simulink model "Clutchless_P2_Parallel"  (R2017b)
settings: Solver=FixedStepAuto  StartTime=0.0  StopTime=length(Speed)  FixedStep=0.01  MaxStep=0.01  RelTol=1e-3  EnableMultiTasking=on
PostLoadFcn:
  | , if any(exist('dsrtsu_mdlpostloadfcn', 'file') == [2, 3, 6]), try dsrtsu_mdlpostloadfcn('Execute', bdroot); catch fprintf('Error in PostLoadFcn (dsrtsu_mdlpostloadfcn) for model "%s":\n %s\n', bdroot, lasterr); end, end,
undefined symbols (not defined in the file): Actuators, APP1_OOR, APP2_OOR, APP_Mismatch, Brk_Flt, cal, Chassis, ClutchEngag, Clutchless_HSC, eng, Engine, EngineTorqueReal, EngOverTemp, ENGTRQ_MSMCH_Degraded_CP, ENGTRQ_MSMCH_ErrCritical_CP, ENGTRQ_MSMCH_LimpHome_CP, EngTrqMismatch, ess, ESSOverTemp, g, gb, Grade, KeyPos_Flt, lib_Actuators, lib_Chassis, lib_Clutchless_HSC, lib_EMachine_2017a, lib_Sensors_2017a, LossCAN, Machine, MCUOverTemp, mot, MotDirMismatch, motor_Trq, MotOverTemp, MotTrqMismatch, mph2ms, PRNDL_Flt, RegenFault, rho, Sensors, t_amb, time, tloop, veh, Vehicle
libraries: simulink x96, EC2_libraries x6, autolibmappedmotor x3, powerlib_meascontrol x2, CalculationGallon x1, lib_DCDC x1, lib_Differential x1, lib_HVESS x1, lib_Engine x1, lib_OBC x1, Scope_new x1, lib_Transmission x1
(part 3 of 10)

== system Clutchless_P2_Parallel/Camaro Plant Model/E-Machine/Soft MCU/Torque Calculation3 ==
  MotTrqReq : Inport
  MotSpd : Inport  Port=2
  MotTrqFdbck : Inport  Port=3
  Voltage : Inport  Port=4
  Abs : Abs  Commented=on  ZeroCross=off
  Abs1 : Abs  Commented=on  ZeroCross=off
  Mapped Generator : autolibmappedmotor/Mapped Motor  port_config=Speed  param_by=Maximum torque and power  w_t=[ 0 375 750 800 ]  T_t=[0.09 0.08 0.07 0]  torque_max=300  power_max=70000  Tc=0.02  param_loss=Tabulated efficiency data  eff=100  w_eff=375  T_eff=0.08  Piron=0  Pbase=0  w_eff_bp=[0 500 1000 1500 2000 2500 3000 3500 4000 4500 5000 5500 6000 6500 7000]  T_eff_bp=[25 50 75 100 112 125 150 165 175 200 225 250 262 275 300]  losses_table=[1.49 1.67 2.21 3.10; 0.42 0.69 1.14 2.03; 0.06 0.24 0.78 1.68; 0.42 0.69 1.14 2.03; 1.49 1.67 2.21 3.10]  efficiency_table=mot.plant.init.geneff_trq.map  J=5e-6  b=1e-5  omega_o=0  T_t_extended=[0 0.07 0.08 0.09 0.08 0.07 0]  w_t_extended=[-800 -750 -375 0 375 750 800]  KLossIron=0  KLossCopper=0  x_w_eff_vec=[-7000 -6500 -6000 -5500 -5000 -4500 -4000 -3500 -3000 -2500 -2000 -1500 -1000 -500 0 500 1000 1500 2000 2500 3000 3500 4000 4500 5000 5500 6000 6500 7000]  x_T_eff_vec=[-300 -275 -262 -250 -225 -200 -175 -165 -150 -125 -112 -100 -75 -50 -25 25 50 75 100 112 125 150 165 175 200 225 250 262 275 300]  x_losses_mat=[2566666.66666667 607894.736842105 517282.051282051 493589.743589743 393750 307317.073170732 233333.333333333 220000 200000 119318.181818182 106909.090909091 95454.5454545455 58333.3333333334 30434.7826086956 213888.888888889 96250 28000 52500 84000 94080 105000 168000 184800 196000 252000 315000 385000 403480 462000 1155000;2383333.33333333 290988.372093023 277232.558139535 221590.909090909 199431.818181818 144444.444444445 98913.0434782608 93260.8695652173 84782.6086956521 70652.1739130434 46468.085106383 41489.3617021276 42391.3043478261 28260.8695652174 198611.111111111 89375 26000 39000 39000 43680 65000 78000 85800 91000 130000 175500 195000 238420 250250 1072500;2200000 183333.333333333 174666.666666667 166666.666666667 150000 76595.744680851 67021.2765957447 63191.4893617021 57446.8085106383 47872.3404255319 42893.6170212766 38297.8723404255 50000 40909.0909090909 183333.333333333 82500 36000 45000 36000 40320 45000 53999.9999999999 59399.9999999999 62999.9999999999 71999.9999999999 135000 150000 157200 165000 990000;2016666.66666667 96542.5531914893 91978.7234042553 87765.9574468085 78989.3617021276 70212.7659574468 61436.1702127659 57925.5319148936 52659.5744680851 43882.9787234042 39319.1489361702 35106.3829787234 45833.3333333334 37500 168055.555555556 75625 33000 41250 33000 36960 41250 49499.9999999999 54449.9999999999 57749.9999999999 65999.9999999999 74249.9999999999 82499.9999999999 86459.9999999999 90749.9999999999 907500;1833333.33333333 87765.9574468085 83617.0212765957 79787.2340425532 71808.5106382979 63829.7872340425 55851.0638297872 52659.5744680851 47872.3404255319 39893.6170212766 35744.6808510638 109756.097560976 41666.6666666667 34090.9090909091 152777.777777778 68750 30000 37500 90000 33600 37500 45000 49499.9999999999 52499.9999999999 59999.9999999999 67499.9999999999 74999.9999999999 78599.9999999999 82499.9999999999 825000;1650000 78989.3617021276 75255.3191489361 71808.5106382979 64627.6595744681 57446.8085106383 50265.9574468085 47393.6170212766 43085.1063829787 35904.2553191489 43826.0869565217 50000 46022.7272727273 36627.9069767442 137500 61875 31500 40500 45000 40320 33750 40500 44550 47250 53999.9999999999 60749.9999999999 67499.9999999999 70739.9999999999 74249.9999999999 742500;1466666.66666667 733333.333333333 698666.666666667 86956.5217391304 57446.8085106383 51063.829787234 44680.8510638298 42127.6595744681 52173.9130434782 43478.2608695652 49777.7777777778 44444.4444444445 48837.2093023256 50000 122222.222222222 55000 40000 42000 40000 44800 40000 48000 39600 42000 48000 53999.9999999999 80000 419200 440000 660000;1283333.33333333 641666.666666667 611333.333333333 97222.2222222223 50265.9574468085 44680.8510638298 53260.8695652174 50217.3913043478 45652.1739130435 48611.1111111111 43555.5555555556 47727.2727272728 57621.9512195122 49358.9743589743 106944.444444444 48125 38500 47250 42000 39200 43750 42000 46200 49000 42000 47250 87500 366800 385000 577500;1100000 550000 524000 500000 75000 38297.8723404255 45652.1739130435 43043.4782608695 39130.4347826087 41666.6666666667 37333.3333333334 33333.3333333334 52777.7777777778 42307.6923076923 91666.6666666667 41250 33000 42750 30000 33600 37500 36000 39600 42000 36000 67500 300000 314400 330000 495000;916666.666666667 458333.333333333 436666.666666667 416666.666666667 375000 333333.333333333 27925.5319148936 35869.5652173913 32608.6956521739 34722.2222222222 31111.1111111111 40697.6744186047 43981.4814814815 39473.6842105263 76388.8888888889 34375 30000 35625 35000 28000 31250 30000 33000 26250 200000 225000 250000 262000 275000 412500;733333.333333333 366666.666666667 349333.333333333 333333.333333333 300000 266666.666666667 233333.333333333 45000 19148.9361702128 27777.7777777778 24888.8888888889 38095.2380952381 35185.1851851852 35135.1351351351 61111.1111111111 27500 26000 28500 32000 22400 25000 18000 39600 140000 160000 180000 200000 209600 220000 330000;550000 275000 262000 250000 225000 200000 175000 15797.8723404255 ...(+5787 chars)]
      settings: SourceProductName=Powertrain Blockset  SourceProductBaseCode=PW
  Mapped Motor : autolibmappedmotor/Mapped Motor  port_config=Speed  param_by=Maximum torque and power  w_t=[ 0 375 750 800 ]  T_t=[0.09 0.08 0.07 0]  torque_max=337  power_max=80000  Tc=0.02  param_loss=Tabulated efficiency data  eff=100  w_eff=375  T_eff=0.08  Piron=0  Pbase=0  w_eff_bp=[0 500 1000 1500 2000 2500 3000 3500 4000 4500 5000 5500 6000 6500 7000]  T_eff_bp="[88.2  98.7 106.4 119 132.2 155.6 175.6 208 243 295.3 328 329 333.5 334.5 335]"  losses_table=[1.49 1.67 2.21 3.10; 0.42 0.69 1.14 2.03; 0.06 0.24 0.78 1.68; 0.42 0.69 1.14 2.03; 1.49 1.67 2.21 3.10]  efficiency_table=mot.plant.init.moteff_trq.map  J=5e-6  b=1e-5  omega_o=0  T_t_extended=[0 0.07 0.08 0.09 0.08 0.07 0]  w_t_extended=[-800 -750 -375 0 375 750 800]  KLossIron=0  KLossCopper=0  x_w_eff_vec=[-7000 -6500 -6000 -5500 -5000 -4500 -4000 -3500 -3000 -2500 -2000 -1500 -1000 -500 0 500 1000 1500 2000 2500 3000 3500 4000 4500 5000 5500 6000 6500 7000]  x_T_eff_vec=[-335 -334.5 -333.5 -329 -328 -295.3 -243 -208 -175.6 -155.6 -132.2 -119 -106.4 -98.7 -88.2 88.2 98.7 106.4 119 132.2 155.6 175.6 208 243 295.3 328 329 333.5 334.5 335]  x_losses_mat=[1563333.33333333 381174.418604651 318340.909090909 314045.454545455 313090.909090909 281877.272727273 231954.545454546 161777.777777778 136577.777777778 94713.0434782608 80469.5652173912 72434.7826086956 31033.3333333334 60078.2608695652 411600 246960 55272 29792 66640 74032 87136 122920 145600 204120 248052 275520 276360 280140 327810 938000;1451666.66666667 296488.636363637 240861.111111111 185956.52173913 185391.304347826 166908.695652174 137347.826086956 117565.217391304 99252.1739130434 87947.8260869565 74721.7391304347 85944.4444444445 94309.090909091 104438.372093023 382200 229320 89817 82992 77350 68744 80912 91312 108160 126360 153556 170560 171080 216775 260910 871000;1340000 273681.818181818 222333.333333333 171652.173913043 171130.434782609 73825.0000000001 126782.608695652 108521.739130435 91617.3913043478 81182.6086956521 68973.9130434782 79333.3333333334 87054.5454545455 96404.6511627907 352800 211680 82908 76608 71400 63456 74688 84288 99840 116640 70872.0000000001 157440 157920 200100 240840 804000;1228333.33333333 1226500 203805.555555556 157347.826086956 115148.936170213 67672.9166666668 55687.5000000001 73021.2765957447 83982.6086956521 74417.3913043478 63226.0869565217 72722.2222222222 79800.0000000001 88370.9302325582 323400 194040 75999 70224 65450 58168 68464 77264 68639.9999999999 53460.0000000001 64966.0000000001 108240 144760 183425 735900 737000;1116666.66666667 1115000 1111666.66666667 182777.777777778 104680.85106383 61520.8333333334 50625.0000000001 66382.9787234042 56042.5531914893 67652.1739130434 57478.2608695652 66111.1111111111 72545.4545454546 80337.2093023256 294000 176400 69090 63840 59500 52880 62240 52679.9999999999 62399.9999999999 48600 59060.0000000001 98399.9999999999 164500 667000 669000 670000;1005000 1003500 1000500 987000 984000 115552.173913043 95086.9565217391 81391.304347826 68713.0434782608 60886.9565217391 66100 59500 65290.9090909091 97496.3414634146 264600 158760 79947 57456 53550 59490 56016 63216 74880 87480 106308 590400 592200 600300 602100 603000;893333.333333333 892000 889333.333333333 877333.333333333 145777.777777778 131244.444444445 84521.7391304347 72347.8260869565 61078.2608695652 54121.7391304347 58755.5555555556 58831.4606741573 69283.7209302326 98700 235200 141120 78960 59584 52360 52880 49792 56192 66560 77760 118120 131200 526400 533600 535200 536000;781666.666666667 780500 778166.666666667 767666.666666667 765333.333333333 689033.333333333 567000 485333.333333333 53443.4782608695 60511.1111111111 57187.6404494382 56795.4545454546 70933.3333333333 97434.6153846153 205800 123480 75999 59584 49980 50897 54460 49168 291200 340200 413420 459200 460600 466900 468300 469000;670000 669000 667000 658000 656000 590600 486000 416000 351200 51866.6666666667 49017.9775280899 58116.2790697675 65378.313253012 93505.2631578948 176400 105840 71064 54264 49980 43626 46680 210720 249600 291600 354360 393600 394800 400200 401400 402000;558333.333333333 557500 555833.333333333 548333.333333333 546666.666666667 492166.666666667 405000 346666.666666667 292666.666666667 259333.333333333 53802.3255813954 56666.6666666667 62395.061728395 110858.695652174 147000 88200 76492.5 50540 47600 46270 155600 175600 208000 243000 295300 328000 329000 333500 334500 335000;446666.666666667 446000 444666.666666667 438666.666666667 437333.333333333 393733.333333333 324000 277333.333333333 234133.333333333 207466.666666667 43041.8604651163 45333.3333333333 60020.5128205128 88686.9565217391 117600 70560 61194 46816 38080 37016 124480 140480 166400 194400 236240 262400 263200 266800 267600 268000;335000 334500 333500 329000 328000 295300 243000 208000 175600 155600 32281.3953488372 34000 50400 79719.2307692308 88200 52920 51817.5 38304 28560 27762 93360 105360 124800 145800 177180 196800 197400 200100 200700 201000;223333.333333333 223000 222333.333333333 219333.333333333 218666.666666667 196866.666666667 162000 138666.666666667 117066.666666667 103733.333333333 21520.9302325581 22666.6666666667 ...(+4913 chars)]
      settings: SourceProductName=Powertrain Blockset  SourceProductBaseCode=PW
  Mapped Motor1 : autolibmappedmotor/Mapped Motor  Commented=on  port_config=Torque  param_by=Maximum torque and power  w_t=[ 0 375 750 800 ]  T_t=[0.09 0.08 0.07 0]  torque_max=337  power_max=70000  Tc=0.02  param_loss=Tabulated efficiency data  eff=100  w_eff=375  T_eff=0.08  Piron=0  Pbase=0  w_eff_bp=[0 500 1000 1500 2000 2500 3000 3500 4000 4500 5000 5500 6000 6500 7000]  T_eff_bp="[88.2  98.7 106.4 119 132.2 155.6 175.6 208 243 295.3 328 329 333.5 334.5 335]"  losses_table=[1.49 1.67 2.21 3.10; 0.42 0.69 1.14 2.03; 0.06 0.24 0.78 1.68; 0.42 0.69 1.14 2.03; 1.49 1.67 2.21 3.10]  efficiency_table=mot.plant.init.moteff_trq.map  J=5e-6  b=1e-5  omega_o=0  T_t_extended=[0 0.07 0.08 0.09 0.08 0.07 0]  w_t_extended=[-800 -750 -375 0 375 750 800]  KLossIron=0  KLossCopper=0  x_w_eff_vec=[-7000 -6500 -6000 -5500 -5000 -4500 -4000 -3500 -3000 -2500 -2000 -1500 -1000 -500 0 500 1000 1500 2000 2500 3000 3500 4000 4500 5000 5500 6000 6500 7000]  x_T_eff_vec=[-335 -334.5 -333.5 -329 -328 -295.3 -243 -208 -175.6 -155.6 -132.2 -119 -106.4 -98.7 -88.2 88.2 98.7 106.4 119 132.2 155.6 175.6 208 243 295.3 328 329 333.5 334.5 335]  x_losses_mat=[1563333.33333333 381174.418604651 318340.909090909 314045.454545455 313090.909090909 281877.272727273 231954.545454546 161777.777777778 136577.777777778 94713.0434782608 80469.5652173912 72434.7826086956 31033.3333333334 60078.2608695652 411600 246960 55272 29792 66640 74032 87136 122920 145600 204120 248052 275520 276360 280140 327810 938000;1451666.66666667 296488.636363637 240861.111111111 185956.52173913 185391.304347826 166908.695652174 137347.826086956 117565.217391304 99252.1739130434 87947.8260869565 74721.7391304347 85944.4444444445 94309.090909091 104438.372093023 382200 229320 89817 82992 77350 68744 80912 91312 108160 126360 153556 170560 171080 216775 260910 871000;1340000 273681.818181818 222333.333333333 171652.173913043 171130.434782609 73825.0000000001 126782.608695652 108521.739130435 91617.3913043478 81182.6086956521 68973.9130434782 79333.3333333334 87054.5454545455 96404.6511627907 352800 211680 82908 76608 71400 63456 74688 84288 99840 116640 70872.0000000001 157440 157920 200100 240840 804000;1228333.33333333 1226500 203805.555555556 157347.826086956 115148.936170213 67672.9166666668 55687.5000000001 73021.2765957447 83982.6086956521 74417.3913043478 63226.0869565217 72722.2222222222 79800.0000000001 88370.9302325582 323400 194040 75999 70224 65450 58168 68464 77264 68639.9999999999 53460.0000000001 64966.0000000001 108240 144760 183425 735900 737000;1116666.66666667 1115000 1111666.66666667 182777.777777778 104680.85106383 61520.8333333334 50625.0000000001 66382.9787234042 56042.5531914893 67652.1739130434 57478.2608695652 66111.1111111111 72545.4545454546 80337.2093023256 294000 176400 69090 63840 59500 52880 62240 52679.9999999999 62399.9999999999 48600 59060.0000000001 98399.9999999999 164500 667000 669000 670000;1005000 1003500 1000500 987000 984000 115552.173913043 95086.9565217391 81391.304347826 68713.0434782608 60886.9565217391 66100 59500 65290.9090909091 97496.3414634146 264600 158760 79947 57456 53550 59490 56016 63216 74880 87480 106308 590400 592200 600300 602100 603000;893333.333333333 892000 889333.333333333 877333.333333333 145777.777777778 131244.444444444 84521.7391304347 72347.8260869565 61078.2608695652 54121.7391304347 58755.5555555556 58831.4606741573 69283.7209302326 98700 235200 141120 78960 59584 52360 52880 49792 56192 66560 77760 118120 131200 526400 533600 535200 536000;781666.666666667 780500 778166.666666667 767666.666666667 765333.333333333 689033.333333333 567000 485333.333333333 53443.4782608695 60511.1111111111 57187.6404494382 56795.4545454546 70933.3333333333 97434.6153846153 205800 123480 75999 59584 49980 50897 54460 49168 291200 340200 413420 459200 460600 466900 468300 469000;670000 669000 667000 658000 656000 590600 486000 416000 351200 51866.6666666667 49017.9775280899 58116.2790697675 65378.313253012 93505.2631578948 176400 105840 71064 54264 49980 43626 46680 210720 249600 291600 354360 393600 394800 400200 401400 402000;558333.333333333 557500 555833.333333333 548333.333333333 546666.666666667 492166.666666667 405000 346666.666666667 292666.666666667 259333.333333333 53802.3255813954 56666.6666666667 62395.061728395 110858.695652174 147000 88200 76492.5 50540 47600 46270 155600 175600 208000 243000 295300 328000 329000 333500 334500 335000;446666.666666667 446000 444666.666666667 438666.666666667 437333.333333333 393733.333333333 324000 277333.333333333 234133.333333333 207466.666666667 43041.8604651163 45333.3333333333 60020.5128205128 88686.9565217391 117600 70560 61194 46816 38080 37016 124480 140480 166400 194400 236240 262400 263200 266800 267600 268000;335000 334500 333500 329000 328000 295300 243000 208000 175600 155600 32281.3953488372 34000 50400 79719.2307692308 88200 52920 51817.5 38304 28560 27762 93360 105360 124800 145800 177180 196800 197400 200100 200700 201000;223333.333333333 223000 222333.333333333 219333.333333333 218666.666666667 196866.666666667 162000 138666.666666667 117066.666666667 103733.333333333 21520.9302325581 22666.6666666667 ...(+4913 chars)]
      settings: SourceProductName=Powertrain Blockset  SourceProductBaseCode=PW
  MinMax : MinMax  Commented=on  Inputs=2  ZeroCross=off
  MotSpd1 : InportShadow  Port=2
  MotTrqReq1 : InportShadow
  Product : Product  Commented=on
  Scope : Scope  Commented=on
  Scope1 : Scope  Commented=on
  Scope2 : Scope  Commented=on
  Sign : Signum  Commented=on  ZeroCross=off
  Subsystem : Subsystem
  Subsystem1 : Subsystem
  Terminator : Terminator
  Terminator1 : Terminator
  Terminator3 : Terminator
  "max torque " : Subsystem  Commented=on
  current : Outport
  mot_trq_out1 : Outport  Port=2
  wires:
  "max torque "/1(max torque) -> Abs1/1
  MotSpd/1 -> "max torque "/2(speed)
  MotTrqReq/1 -> Sign/1, Abs/1, "max torque "/1(Req)
  Sign/1 -> Product/1
  MinMax/1 -> Product/2
  Abs/1 -> MinMax/1
  Abs1/1 -> MinMax/2
  MotTrqFdbck/1 -> "max torque "/3(torque)
  MotTrqReq1/1 -> Mapped Generator/3, Subsystem1/2(In2), Subsystem/2(In2), Mapped Motor1/2, Mapped Motor/3
  MotSpd1/1 -> Mapped Generator/2, Mapped Motor/2
  Voltage/1 -> Mapped Motor1/1, Mapped Generator/1, Mapped Motor/1
  Mapped Motor/1 -> Terminator/1
  Mapped Generator/1 -> Terminator1/1
  Mapped Motor/3 -> Subsystem/1(In1)
  Mapped Generator/3 -> Subsystem/3(In3)
  Mapped Motor/2 -> Subsystem1/1(In1)
  Mapped Generator/2 -> Subsystem1/3(In3)
  Subsystem/1(Torq) -> mot_trq_out1/1
  Subsystem1/1(Current) -> current/1
  Mapped Motor1/3 -> Scope1/1
  Mapped Motor1/2 -> Scope2/1
  Mapped Motor1/1 -> Terminator3/1
  Mapped Motor1/4 -> Scope/1

== system Clutchless_P2_Parallel/Camaro Plant Model/Scopes/AxlTrq_to_EngTrq2/Ratio Filter ==
  Ratio : Inport
  Abs : Abs
  Compare To Zero : simulink/Logic and Bit Operations/Compare To Zero  relop===  OutDataTypeStr=boolean
  Constant : Constant  Value=cal.Time.TrnsOvrllEstTrqRatioSwitch
  Mature_Delay : EC2_libraries/Mature_Delay
      settings: SourceProductName=The database C:\Users\vrajm\AppData\Roaming\MathWorks\MATLAB\R2017b\slblocks_master.db is locked, or a table in the database is locked. (database is locked)
  Memory1 : Memory  InitialCondition=1
  Switch1 : Switch  Threshold=1
  Switch2 : Switch  Threshold=1
  Filtered_Ratio : Outport
  wires:
  Ratio/1 -> Compare To Zero/1, Abs/1
  Compare To Zero/1 -> Mature_Delay/1, Switch2/2
  Abs/1 -> Switch1/1, Switch2/3
  Switch1/1 -> Switch2/1
  Constant/1 -> Mature_Delay/2
  Mature_Delay/1 -> Switch1/2
  Memory1/1 -> Switch1/3
  Switch2/1 -> Filtered_Ratio/1, Memory1/1  "gear_ratio"

== system Clutchless_P2_Parallel/Camaro Plant Model/Scopes/AxlTrq_to_MtrTrq2/Ratio Filter ==
  Ratio : Inport
  Abs : Abs
  Compare To Zero : simulink/Logic and Bit Operations/Compare To Zero  relop===  OutDataTypeStr=boolean
  Constant : Constant  Value=cal.Time.TrnsOvrllEstTrqRatioSwitch
  Mature_Delay : EC2_libraries/Mature_Delay
      settings: SourceProductName=The database C:\Users\vrajm\AppData\Roaming\MathWorks\MATLAB\R2017b\slblocks_master.db is locked, or a table in the database is locked. (database is locked)
  Memory1 : Memory  InitialCondition=1
  Switch1 : Switch  Threshold=1
  Switch2 : Switch  Threshold=1
  Filtered_Ratio : Outport
  wires:
  Ratio/1 -> Compare To Zero/1, Abs/1
  Compare To Zero/1 -> Mature_Delay/1, Switch2/2
  Abs/1 -> Switch1/1, Switch2/3
  Switch1/1 -> Switch2/1
  Constant/1 -> Mature_Delay/2
  Mature_Delay/1 -> Switch1/2
  Memory1/1 -> Switch1/3
  Switch2/1 -> Filtered_Ratio/1, Memory1/1  "gear_ratio"

== system Clutchless_P2_Parallel/Clutchless_HSC/HSC/Camaro Fault Detection/Component Diagnostic ==
  note: Component Status Setting Rule
      | xxx_CompStatus could be 0, 1, 2 or 3
      | 0: component needs to be offline
      | 1: component needs torque plant to deliver creep torque
      | 2: component needs torque plant to limit maximum torque delivery
      | 3: component needs torque plant to operate normally
  note: Component Diagnostics
  SignalDiag : Inport
  Bus Creator : BusCreator  Inputs=6
  Driver Input Diagnostic : Subsystem
  ESS Component Diagnostic : Subsystem
  Engine Component Diagnostic : Subsystem
  Override Driver Status : Subsystem
  Override ESS Status : Subsystem
  Override Engine Status : Subsystem
  Override TCM Status : Subsystem
  Transmission Component Diagnostic : Subsystem
  CompDiag : Outport
  wires:
  SignalDiag/1 -> Engine Component Diagnostic/1(In1), Transmission Component Diagnostic/1(In1), Bus Creator/6, ESS Component Diagnostic/1(In1), Driver Input Diagnostic/1(In1)  "RawSig"
  Bus Creator/1 -> CompDiag/1
  Driver Input Diagnostic/1(Out1) -> Override Driver Status/1(In1)  "Diver_CompDiag"
  ESS Component Diagnostic/1(Out1) -> Override ESS Status/1(In1)  "ESS_CompDiag"
  Engine Component Diagnostic/1(Out1) -> Override Engine Status/1(In1)  "ECM_CompDiag"
  Transmission Component Diagnostic/1(Out1) -> Override TCM Status/1(In1)  "TCM_CompDiag"
  Override ESS Status/1(Out1) -> Bus Creator/2  "BMS_Status"
  Override Engine Status/1(Out1) -> Bus Creator/3  "ECM_Status"
  Override TCM Status/1(Out1) -> Bus Creator/5  "TCM_Status"
  Override Driver Status/1(Out1) -> Bus Creator/1  "Driver_Input_Status"
  Engine Component Diagnostic/2(Out2) -> Bus Creator/4  "EngTrqMismchType"

== system Clutchless_P2_Parallel/Clutchless_HSC/HSC/Camaro Fault Detection/Input Conversions ==
  note: Input Conversions and Override Switches
  note: These subsystems convert variable types to match those used in the
      | supervisor. In addition, override switches installed on each signal can
      | be used to manually override and signal for testing purposes
  RawSig : Inport
  BMS_Conversions : Subsystem
  Bus Creator : BusCreator  Inputs=5
  DriverInput_Conversions : Subsystem
  ECM_Conversions : Subsystem
  TCM_Conversions : Subsystem
  VehSig : Outport
  wires:
  DriverInput_Conversions/1(Out1) -> Bus Creator/1
  Bus Creator/1 -> VehSig/1  "InputConvAndOvrd"
  BMS_Conversions/1(Out1) -> Bus Creator/2
  RawSig/1 -> DriverInput_Conversions/1(In1), Bus Creator/5, TCM_Conversions/1(In1), ECM_Conversions/1(In1), BMS_Conversions/1(In1)  "RawSig"
  ECM_Conversions/1(Out1) -> Bus Creator/3
  TCM_Conversions/1(Out1) -> Bus Creator/4

== system Clutchless_P2_Parallel/Clutchless_HSC/HSC/Camaro Fault Detection/Signal Diagnostic ==
  note: These subsystems evaluate each signal for proper value range and other checks
  note: Signal Diagnostics
  VehSig : Inport
  Bus Creator : BusCreator  Inputs=5
  Driver Signal Diagnostic : Subsystem
  ESS Signal Diagnostic : Subsystem
  Engine Signal Diagnostic : Subsystem
  Subsystem1 : Subsystem
      mask Display: fprintf('Signal Naming Rule')
  Transmission Signal Diagnostic : Subsystem
  SignalDiag : Outport
  wires:
  VehSig/1 -> ESS Signal Diagnostic/1(Sensors1), Driver Signal Diagnostic/1(Sensors1), Engine Signal Diagnostic/1(Sensors1), Bus Creator/5, Transmission Signal Diagnostic/1(Sensors1)
  Driver Signal Diagnostic/1(Driver_SigDiag) -> Bus Creator/1  "Driver_SigDiag"
  ESS Signal Diagnostic/1(ESS_SigDiag) -> Bus Creator/2  "ESS_SigDiag"
  Engine Signal Diagnostic/1(Engine_SigDiag) -> Bus Creator/3  "Engine_SigDiag"
  Transmission Signal Diagnostic/1(Out2) -> Bus Creator/4  "Transmission_SigDiag"
  Bus Creator/1 -> SignalDiag/1  "SignalDiag"

== system Clutchless_P2_Parallel/Clutchless_HSC/HSC/Driver_Requests/APP_BPP to DrvIntndAxlTrq2 ==
  note: $Author: fy6949 $
      | $Rev: 577 $
      | $Date: 2017-1-19 08:53:15 -0500  $
  note: Note:Driver requested Axle Torque Calculation
  Sensors : Inport
  Diag : Inport  Port=2
  Controls : Inport  Port=3
  Bus Selector : BusSelector  OutputSignals=from_Analog.Driver_APP1,from_CAN.fromVEH_CAN.from_BCM.BrkPdlPos,from_CAN.fromEBCAN.from_ECM.VehSpdAvgDrvn,from_CAN.fromVEH_CAN.from_TCM.TrnGrRat,from_CAN.fromHV_CAN.from_MCU.INV_VCU_01.INV_Speed
  Bus Selector1 : BusSelector  OutputSignals=CompSig.RawSig.Driver_SigDiag.Drv_APP_Agree
  Bus Selector2 : BusSelector  OutputSignals=mode
  Post Driver Intnded Axle Torque : Subsystem
  Terminator : Terminator
  Terminator1 : Terminator
  IntndAxlTrq : Outport
  wires:
  Bus Selector2/1 -> Post Driver Intnded Axle Torque/5(Mode)  "<mode>"
  Bus Selector1/1 -> Terminator1/1  "<Drv_APP_Agree>"
  Diag/1 -> Bus Selector1/1
  Post Driver Intnded Axle Torque/2(BrkIntndAxlTrq) -> Terminator/1
  Bus Selector/1 -> Post Driver Intnded Axle Torque/1(APP)  "<Driver_APP1>"
  Bus Selector/4 -> Post Driver Intnded Axle Torque/4(TransGearRatio)  "<TrnGrRat>"
  Bus Selector/5 -> Post Driver Intnded Axle Torque/6(Motor_Speed)  "<INV_Speed>"
  Bus Selector/3 -> Post Driver Intnded Axle Torque/3(VehicleSpeed)  "<VehSpdAvgDrvn>"
  Bus Selector/2 -> Post Driver Intnded Axle Torque/2(BPP)  "<BrkPdlPos>"
  Post Driver Intnded Axle Torque/1(IntndAxlTrq) -> IntndAxlTrq/1
  Controls/1 -> Bus Selector2/1
  Sensors/1 -> Bus Selector/1

== system Clutchless_P2_Parallel/Clutchless_HSC/HSC/Powertrain Manager/HV Manager ==
  Sensors : Inport
  Controls : Inport  Port=2
  Axiomatic_Output_Manager : Subsystem
  BMS_Manager : Subsystem
  Bus Creator1 : BusCreator  Inputs=4
  DCDC Manager : Subsystem
  Inverter Manager : Subsystem
  OBC_Manager : Subsystem
  BMS_CAN : Outport
  HV_BUS_Status : Outport  Port=2
  OBC_CAN : Outport  Port=3
  OBC_Digital : Outport  Port=4
  BMS_Digital : Outport  Port=5
  Axiomatic_CAN : Outport  Port=6
  tag scope: MCU_CAN=global
  wires:
  [MCU_Status] -> BMS_Manager/3(In1)
  DCDC Manager/1(Out1) -> Bus Creator1/4
  Inverter Manager/3(MCU_Relay) -> Bus Creator1/3  "MCU_Relay"
  Axiomatic_Output_Manager/1(Axiomatic_CAN) -> Axiomatic_CAN/1
  BMS_Manager/3(BMS Digital) -> BMS_Digital/1
  BMS_Manager/1(BMS CAN) -> BMS_CAN/1
  Controls/1 -> Inverter Manager/3(Control), DCDC Manager/3(In2), DCDC Manager/2(In1), BMS_Manager/2(Controls)
  OBC_Manager/2(OBC_Digital) -> OBC_Digital/1
  OBC_Manager/1(OBC CAN) -> OBC_CAN/1
  [HV_BUS_Status] -> OBC_Manager/1(HV_Status)
  BMS_Manager/2(HV_BUS_Status) -> HV_BUS_Status/1, [HV_BUS_Status]  "HV_BUS_Status"
  [HV_BUS_Status] -> Axiomatic_Output_Manager/2(HV_Bus_Status)
  [HV_BUS_Status] -> Inverter Manager/1(HV_Bus_Status)  "HV_BUS_Status"
  Sensors/1 -> Inverter Manager/2(Sensors), OBC_Manager/2(Sensors), Axiomatic_Output_Manager/1(Sensors), DCDC Manager/1(BMSInput), BMS_Manager/1(Sensors)
  Inverter Manager/1(MCU_Status) -> Bus Creator1/1, [MCU_Status]  "MCU_Status"
  Inverter Manager/2(MCU_CAN) -> Bus Creator1/2  "MCU_CAN"
  Bus Creator1/1 -> [MCU_CAN]

== system Clutchless_P2_Parallel/Clutchless_HSC/HSC/Powertrain Manager/Output Conversion ==
  In1 : Inport
  In2 : Inport  Port=2
  In3 : Inport  Port=3
  In4 : Inport  Port=4
  In5 : Inport  Port=5
  In8 : Inport  Port=6
  In9 : Inport  Port=7
  In10 : Inport  Port=8
  In11 : Inport  Port=9
  Bus Creator : BusCreator  Inputs=14
  Bus Creator1 : BusCreator  Inputs=9
  Bus Selector2 : BusSelector  OutputSignals=powerMode,EnablePrplsn,ClutchEngage,EngAppReq,EngOnReq,MtrTrqCmd,EnableInverter,EngTrqCmd,HV_req,SysPwrMd_0_3,TransShftLvrPos,VehSpdAvgDrvn_kph,AccPos_Perc,SportsModeEnable
  Data Type Conversion{,2..3,5..13} (12 alike) : DataTypeConversion
  Memory : Memory
  Out1 : Outport
  wires:
  Bus Selector2/14 -> Bus Creator/14  "<SportsModeEnable>"
  In11/1 -> Bus Creator1/9
  In4/1 -> Bus Selector2/1
  Bus Selector2/1 -> Memory/1  "<powerMode>"
  Bus Selector2/2 -> Data Type Conversion2/1  "<EnablePrplsn>"
  Bus Selector2/3 -> Data Type Conversion3/1  "<ClutchEngage>"
  Bus Selector2/5 -> Data Type Conversion5/1  "<EngOnReq>"
  Bus Selector2/6 -> Data Type Conversion6/1  "<MtrTrqCmd>"
  Bus Selector2/7 -> Data Type Conversion7/1  "<EnableInverter>"
  Bus Selector2/8 -> Data Type Conversion8/1  "<EngTrqCmd>"
  Bus Selector2/9 -> Data Type Conversion9/1  "<HV_req>"
  Bus Selector2/10 -> Data Type Conversion10/1  "<SysPwrMd_0_3>"
  Data Type Conversion2/1 -> Bus Creator/2  "EnablePrplsn"
  Data Type Conversion3/1 -> Bus Creator/3  "ClutchEngage"
  Bus Selector2/4 -> Bus Creator/4  "<EngAppReq>"
  Data Type Conversion6/1 -> Bus Creator/6  "Torque_Command"
  Data Type Conversion7/1 -> Bus Creator/7  "Inverter_Enable"
  Data Type Conversion8/1 -> Bus Creator/8  "EngTrqCmd"
  Data Type Conversion9/1 -> Bus Creator/9  "HV_req"
  Data Type Conversion10/1 -> Bus Creator/10  "SysPwrMd"
  Data Type Conversion/1 -> Bus Creator/1  "powerMode"
  Data Type Conversion5/1 -> Bus Creator/5  "EngOnReq"
  Bus Creator1/1 -> Out1/1
  In1/1 -> Bus Creator1/1
  In2/1 -> Bus Creator1/2
  In3/1 -> Bus Creator1/3
  Bus Creator/1 -> Bus Creator1/4  "Controls"
  In5/1 -> Bus Creator1/5
  Bus Selector2/11 -> Data Type Conversion11/1  "<TransShftLvrPos>"
  Data Type Conversion11/1 -> Bus Creator/11  "ShftLvrPos"
  Bus Selector2/12 -> Data Type Conversion12/1  "<VehSpdAvgDrvn_kph>"
  Data Type Conversion12/1 -> Bus Creator/12  "VehSpdAvgDrvn_kph"
  Bus Selector2/13 -> Data Type Conversion13/1  "<AccPos_Perc>"
  Data Type Conversion13/1 -> Bus Creator/13  "AccPos_Perc"
  Memory/1 -> Data Type Conversion/1
  In8/1 -> Bus Creator1/6
  In9/1 -> Bus Creator1/7
  In10/1 -> Bus Creator1/8

== system Clutchless_P2_Parallel/Clutchless_HSC/HSC/Powertrain Manager/Thermal Manager ==
  In2 : Inport
  Bus Creator : BusCreator  Inputs=3
  Bus Creator1 : BusCreator  Inputs=4
  Bus Creator2 : BusCreator  Inputs=4
  Bus Creator3 : BusCreator  Inputs=3
  Bus Creator4 : BusCreator  Inputs=1
  Bus Selector : BusSelector  OutputSignals=from_CAN.fromEBCAN.from_ECM.EngCltTmp,from_CAN.fromHV_CAN.from_BMSHybrid.BMS_Temperatur,from_CAN.fromHV_CAN.from_MCU.INV_VCU_04.INV_InverterTemperature,from_CAN.fromHV_CAN.from_MCU.INV_VCU_04.INV_ElectricMachineTemperature,from_CAN.fromEBCAN.from_ECM.EngRunAtv,from_CAN.fromHV_CAN.from_BMSHybrid.BMS_HYB_02.BMS_IstModus,from_CAN.fromVEH_CAN.from_BCM.SysPwrMd,from_CAN.fromEBCAN.from_ECM.VehSpdAvgDrvn
  Bus Selector3 : BusSelector  OutputSignals=from_CAN.fromHV_CAN.from_BMSHybrid.BMS_HYB_02.BMS_Fehler_Pilot
  Compare To Constant1 : simulink/Logic and Bit Operations/Compare To Constant  relop=>  const=0  OutDataTypeStr=boolean
  Cooling Fan Manger : Subsystem
  Data Type Conversion : DataTypeConversion  OutDataTypeStr=double
  ESS Pump Manger : Subsystem
  MotInv Pump Manger : Subsystem
  Out1 : Outport
  wires:
  Compare To Constant1/1 -> Data Type Conversion/1
  Data Type Conversion/1 -> Bus Creator4/1  "FuelPump_Disable"
  Bus Creator4/1 -> Bus Creator1/4  "Pump_Commands"
  Bus Selector3/1 -> Compare To Constant1/1  "<BMS_Fehler_Pilot>"
  In2/1 -> Bus Selector/1, Bus Selector3/1
  Bus Creator3/1 -> Bus Creator/2  "Component_State"
  Bus Creator2/1 -> Bus Creator/1  "Temp_Signals"
  MotInv Pump Manger/1(MotInvpump_control) -> Bus Creator1/3  "MotMCU_Pump_Control"
  ESS Pump Manger/1(ESS_Thermal_Control) -> Bus Creator1/2  "ESS_Pump_Control"
  Bus Creator/1 -> MotInv Pump Manger/1(MotInv_temp), ESS Pump Manger/1(ESS_temp), Cooling Fan Manger/1(Temp)
  Cooling Fan Manger/1(Fan_control) -> Bus Creator1/1  "Fan_Control"
  Bus Creator1/1 -> Out1/1  "Thermal_Control"
  Bus Selector/1 -> Bus Creator2/1  "<EngCltTmp>"
  Bus Selector/2 -> Bus Creator2/2  "<BMS_Temperatur>"
  Bus Selector/3 -> Bus Creator2/3  "<INV_InverterTemperature>"
  Bus Selector/4 -> Bus Creator2/4  "<INV_ElectricMachineTemperature>"
  Bus Selector/5 -> Bus Creator3/1  "<EngRunAtv>"
  Bus Selector/6 -> Bus Creator3/2  "<BMS_IstModus>"
  Bus Selector/7 -> Bus Creator3/3  "<SysPwrMd>"
  Bus Selector/8 -> Bus Creator/3  "<VehSpdAvgDrvn>"
